simulink model "six_plus_six_AcmsteeringV09_main"  (R2014a)
settings: Solver=FixedStepDiscrete  StartTime=0.0  StopTime=10.0  FixedStep=0.0005  RelTol=1e-3
InitFcn:
  | Veh_Par_wxt
values from neighbouring files (symbols this model uses):
  acc_spdctl = [0 100]    [Veh_Par_wxt.m]
  ag_thr = ecucoder_cal(ag_thr)    [Veh_Par_wxt.m]
  B = 1.8    [Veh_Par_wxt.m]
  bra_em = 100    [Veh_Par_wxt.m]
  bra_pre_gz2 = 100/3    (= 33.3333333333)    [Veh_Par_wxt.m]
  bra_pre_gz34 = 10/3    (= 3.33333333333)    [Veh_Par_wxt.m]
  bra_pre_yd = 10/2    (= 5)    [Veh_Par_wxt.m]
  brakepre_dem_data = [0 1 2 3 4 5 6 7 8 9 10]    [Veh_Par_wxt.m]
  brakeTrq_dem_data = [0 125 251 376 502 627 753 878 1004 1129 1255]    [Veh_Par_wxt.m]
  bratrq_max = 4*1255    (= 5020)    [Veh_Par_wxt.m]
  eff_tran = 0.9    [Veh_Par_wxt.m]
  ESP_switch = ecucoder_cal(ESP_switch)    [Veh_Par_wxt.m]
  G = Mass*g    (= 15696)    [Veh_Par_wxt.m]
  kd1 = ecucoder_cal(kd1)    [Veh_Par_wxt.m]
  kd2 = 0    [Veh_Par_wxt.m]
  ki1 = ecucoder_cal(ki1)    [Veh_Par_wxt.m]
  ki2 = 1    [Veh_Par_wxt.m]
  kp1 = ecucoder_cal(kp1)    [Veh_Par_wxt.m]
  kp2 = 300    [Veh_Par_wxt.m]
  L = L1+L2    (= 2.9)    [Veh_Par_wxt.m]
  premax = 100    [Veh_Par_wxt.m]
  Radius = 0.4572/2    (= 0.2286)    [Veh_Par_wxt.m]
  RC_switch = ecucoder_cal(RC_switch)    [Veh_Par_wxt.m]
  s_opt_yi = 0.15    [Veh_Par_wxt.m]
  s_opt_zhuan = 0.8    [Veh_Par_wxt.m]
  s_opt_zhuan_add = 0.05    [Veh_Par_wxt.m]
  s_opt_zhuan_table = [0.8 0.8 0.3 0.3]    [Veh_Par_wxt.m]
  spd_map_mot = [0 499.85 999.79 1500 2000 2500 3000 3500 4000 4500 4999.8 5999.8]    [Veh_Par_wxt.m]
  spd_spdctl = [0 500]    [Veh_Par_wxt.m]
  speed_thr_park = 5/3.6/Radius*tras_ratio*30/pi    (= 464.143899364)    [Veh_Par_wxt.m]
  TCS_switch = ecucoder_cal(TCS_switch)    [Veh_Par_wxt.m]
  tras_ratio = 8    [Veh_Par_wxt.m]
  trq_map_mot = [70.5 70.012 71.154 65.797 53.917 45.159 38.073 32.685 27.48 17.133 14.949 10.07]    [Veh_Par_wxt.m]
  trqmax_yd = 70.5    [Veh_Par_wxt.m]
  trqmax_zx = 70.5    [Veh_Par_wxt.m]
  trqmaxneg = -70.5    [Veh_Par_wxt.m]
  v_gain = 0.9    [Veh_Par_wxt.m]
  v_table = [0 5 20 100]    [Veh_Par_wxt.m]
  v_thr_park = 5    [Veh_Par_wxt.m]
  zhidong_bianmazhi = [-140000 750000]    [Veh_Par_wxt.m]
  zhidong_down = -140000    [Veh_Par_wxt.m]
  zhidong_up = 750000    [Veh_Par_wxt.m]
  zhidong_youmen = [0 100]    [Veh_Par_wxt.m]
  zhuanxiang_bianmazhi = [-400000 0 400000]    [Veh_Par_wxt.m]
  zhuanxiang_down = -400000    [Veh_Par_wxt.m]
  zhuanxiang_up = 400000    [Veh_Par_wxt.m]
  zhuanxiang_youmen = [-100 0 100]    [Veh_Par_wxt.m]
undefined symbols (not defined in the file or in its folder): ecucoder_acal, guzhang_lf, guzhang_lm, guzhang_lr, guzhang_rf, guzhang_rm, guzhang_rr, myFIS
libraries: simulink x979, ec5744lib x59, fuzblock x2
(part 15 of 26)

== system six_plus_six_AcmsteeringV09_main/MainControl/mode_control/center_steer ==
  Signals : Inport
  Action Port : ActionPort  ActionType=case
  Mux : Mux  Inputs=10
  center_steer : Subsystem
  center_steer_dem : Outport
  wires:
  Mux/1 -> center_steer_dem/1
  Signals/1 -> center_steer/1(Signals)
  center_steer/6(mot_rr) -> Mux/6
  center_steer/1(mot_lf) -> Mux/1
  center_steer/4(mot_rf) -> Mux/4
  center_steer/3(mot_lr) -> Mux/3
  center_steer/5(mot_rm) -> Mux/5
  center_steer/2(mot_lm) -> Mux/2
  center_steer/7(motec_position_1) -> Mux/7
  center_steer/8(motec_position_2) -> Mux/8
  center_steer/10(motec_position_4) -> Mux/10
  center_steer/9(motec_position_3) -> Mux/9

== system six_plus_six_AcmsteeringV09_main/MainControl/mode_control/emergency_stop ==
  Signals : Inport
  Action Port : ActionPort  ActionType=case
  Mux : Mux  Inputs=10
  emergency_stop : Subsystem
  emergency_stop_dem : Outport
  wires:
  Mux/1 -> emergency_stop_dem/1
  Signals/1 -> emergency_stop/1(Signals)
  emergency_stop/8(motec_position_2) -> Mux/8
  emergency_stop/9(motec_position_3) -> Mux/9
  emergency_stop/10(motec_position_4) -> Mux/10
  emergency_stop/7(motec_position_1) -> Mux/7
  emergency_stop/3(mot_lr) -> Mux/3
  emergency_stop/1(mot_lf) -> Mux/1
  emergency_stop/2(mot_lm) -> Mux/2
  emergency_stop/5(mot_rm) -> Mux/5
  emergency_stop/6(mot_rr) -> Mux/6
  emergency_stop/4(mot_rf) -> Mux/4

== system six_plus_six_AcmsteeringV09_main/MainControl/mode_control/forward ==
  Signals : Inport
  Action Port : ActionPort  ActionType=case
  forward : Subsystem
  forward_dem : Outport
  wires:
  Signals/1 -> forward/1(Signals)
  forward/1(forward_dem) -> forward_dem/1

== system six_plus_six_AcmsteeringV09_main/MainControl/mode_control/neutral ==
  Signals : Inport
  Action Port : ActionPort  ActionType=case
  Mux : Mux  Inputs=10
  neutral : Subsystem
  neutral_dem : Outport
  wires:
  Mux/1 -> neutral_dem/1
  Signals/1 -> neutral/1(Signals)
  neutral/3(mot_lr) -> Mux/3
  neutral/5(mot_rm) -> Mux/5
  neutral/6(mot_rr) -> Mux/6
  neutral/2(mot_lm) -> Mux/2
  neutral/1(mot_lf) -> Mux/1
  neutral/4(mot_rf) -> Mux/4
  neutral/7(motec_position_1) -> Mux/7
  neutral/8(motec_position_2) -> Mux/8
  neutral/10(motec_position_4) -> Mux/10
  neutral/9(motec_position_3) -> Mux/9

== system six_plus_six_AcmsteeringV09_main/Subsystem/VCU1/VCU1_CtrlModel ==
  VCU1_CtrlModel : Inport
  Constant{2..8} (7 alike) : Constant  Value=0  OutDataTypeStr=uint8
  VCU1_CtrlModelRon : Rounding  Operator=round
  VCU1_CtrlModel_1sat : Saturate  UpperLimit=4  LowerLimit=0
  VCU1_CtrlModel_Convert : DataTypeConversion  OutDataTypeStr=uint8
  VCU1_CtrlModel_Convert1 : DataTypeConversion  OutDataTypeStr=uint32
  VCU1_CtrlModel_D : Product  Inputs=*/
  VCU1_CtrlModel_F : Constant  OutDataTypeStr=single
  VCU1_CtrlModel_L : simulink/Logic and Bit Operations/Bitwise Operator  logicop=AND  UseBitMask=on  BitMask=4  BitMaskRealWorld=Stored Integer
  VCU1_CtrlModel_O : Constant  Value=0  OutDataTypeStr=single
  VCU1_CtrlModel_S : ArithShift  BitShiftNumber=-2
  VCU1_CtrlModel_sat : Saturate  UpperLimit=1  LowerLimit=0
  VCU1_CtrlModel_st : Sum  Inputs=+-
  output1 : Outport
  output2 : Outport  Port=2
  output3 : Outport  Port=3
  output4 : Outport  Port=4
  output5 : Outport  Port=5
  output6 : Outport  Port=6
  output7 : Outport  Port=7
  output8 : Outport  Port=8
  wires:
  VCU1_CtrlModel/1 -> VCU1_CtrlModel_sat/1
  VCU1_CtrlModel_sat/1 -> VCU1_CtrlModel_st/1
  VCU1_CtrlModel_O/1 -> VCU1_CtrlModel_st/2
  VCU1_CtrlModel_st/1 -> VCU1_CtrlModel_D/1
  VCU1_CtrlModel_F/1 -> VCU1_CtrlModel_D/2
  VCU1_CtrlModel_D/1 -> VCU1_CtrlModelRon/1
  VCU1_CtrlModelRon/1 -> VCU1_CtrlModel_S/1
  VCU1_CtrlModel_S/1 -> VCU1_CtrlModel_1sat/1
  VCU1_CtrlModel_1sat/1 -> VCU1_CtrlModel_Convert1/1
  VCU1_CtrlModel_Convert1/1 -> VCU1_CtrlModel_L/1
  VCU1_CtrlModel_L/1 -> VCU1_CtrlModel_Convert/1
  VCU1_CtrlModel_Convert/1 -> output1/1
  Constant2/1 -> output2/1
  Constant3/1 -> output3/1
  Constant4/1 -> output4/1
  Constant5/1 -> output5/1
  Constant6/1 -> output6/1
  Constant7/1 -> output7/1
  Constant8/1 -> output8/1

== system six_plus_six_AcmsteeringV09_main/Subsystem/VCU1/VCU1_EnableReq ==
  VCU1_EnableReq : Inport
  Constant{2..8} (7 alike) : Constant  Value=0  OutDataTypeStr=uint8
  VCU1_EnableReqRon : Rounding  Operator=round
  VCU1_EnableReq_1sat : Saturate  UpperLimit=3  LowerLimit=0
  VCU1_EnableReq_Convert : DataTypeConversion  OutDataTypeStr=uint8
  VCU1_EnableReq_Convert1 : DataTypeConversion  OutDataTypeStr=uint32
  VCU1_EnableReq_D : Product  Inputs=*/
  VCU1_EnableReq_F : Constant  OutDataTypeStr=single
  VCU1_EnableReq_L : simulink/Logic and Bit Operations/Bitwise Operator  logicop=AND  UseBitMask=on  BitMask=3  BitMaskRealWorld=Stored Integer
  VCU1_EnableReq_O : Constant  Value=0  OutDataTypeStr=single
  VCU1_EnableReq_S : ArithShift
  VCU1_EnableReq_sat : Saturate  UpperLimit=3  LowerLimit=0
  VCU1_EnableReq_st : Sum  Inputs=+-
  output1 : Outport
  output2 : Outport  Port=2
  output3 : Outport  Port=3
  output4 : Outport  Port=4
  output5 : Outport  Port=5
  output6 : Outport  Port=6
  output7 : Outport  Port=7
  output8 : Outport  Port=8
  wires:
  VCU1_EnableReq/1 -> VCU1_EnableReq_sat/1
  VCU1_EnableReq_sat/1 -> VCU1_EnableReq_st/1
  VCU1_EnableReq_O/1 -> VCU1_EnableReq_st/2
  VCU1_EnableReq_st/1 -> VCU1_EnableReq_D/1
  VCU1_EnableReq_F/1 -> VCU1_EnableReq_D/2
  VCU1_EnableReq_D/1 -> VCU1_EnableReqRon/1
  VCU1_EnableReqRon/1 -> VCU1_EnableReq_S/1
  VCU1_EnableReq_S/1 -> VCU1_EnableReq_1sat/1
  VCU1_EnableReq_1sat/1 -> VCU1_EnableReq_Convert1/1
  VCU1_EnableReq_Convert1/1 -> VCU1_EnableReq_L/1
  VCU1_EnableReq_L/1 -> VCU1_EnableReq_Convert/1
  VCU1_EnableReq_Convert/1 -> output1/1
  Constant2/1 -> output2/1
  Constant3/1 -> output3/1
  Constant4/1 -> output4/1
  Constant5/1 -> output5/1
  Constant6/1 -> output6/1
  Constant7/1 -> output7/1
  Constant8/1 -> output8/1

== system six_plus_six_AcmsteeringV09_main/Subsystem/VCU1/VCU1_GearCmd ==
  VCU1_GearCmd : Inport
  Constant{2..8} (7 alike) : Constant  Value=0  OutDataTypeStr=uint8
  VCU1_GearCmdRon : Rounding  Operator=round
  VCU1_GearCmd_1sat : Saturate  UpperLimit=24  LowerLimit=0
  VCU1_GearCmd_Convert : DataTypeConversion  OutDataTypeStr=uint8
  VCU1_GearCmd_Convert1 : DataTypeConversion  OutDataTypeStr=uint32
  VCU1_GearCmd_D : Product  Inputs=*/
  VCU1_GearCmd_F : Constant  OutDataTypeStr=single
  VCU1_GearCmd_L : simulink/Logic and Bit Operations/Bitwise Operator  logicop=AND  UseBitMask=on  BitMask=24  BitMaskRealWorld=Stored Integer
  VCU1_GearCmd_O : Constant  Value=0  OutDataTypeStr=single
  VCU1_GearCmd_S : ArithShift  BitShiftNumber=-3
  VCU1_GearCmd_sat : Saturate  UpperLimit=3  LowerLimit=0
  VCU1_GearCmd_st : Sum  Inputs=+-
  output1 : Outport
  output2 : Outport  Port=2
  output3 : Outport  Port=3
  output4 : Outport  Port=4
  output5 : Outport  Port=5
  output6 : Outport  Port=6
  output7 : Outport  Port=7
  output8 : Outport  Port=8
  wires:
  VCU1_GearCmd/1 -> VCU1_GearCmd_sat/1
  VCU1_GearCmd_sat/1 -> VCU1_GearCmd_st/1
  VCU1_GearCmd_O/1 -> VCU1_GearCmd_st/2
  VCU1_GearCmd_st/1 -> VCU1_GearCmd_D/1
  VCU1_GearCmd_F/1 -> VCU1_GearCmd_D/2
  VCU1_GearCmd_D/1 -> VCU1_GearCmdRon/1
  VCU1_GearCmdRon/1 -> VCU1_GearCmd_S/1
  VCU1_GearCmd_S/1 -> VCU1_GearCmd_1sat/1
  VCU1_GearCmd_1sat/1 -> VCU1_GearCmd_Convert1/1
  VCU1_GearCmd_Convert1/1 -> VCU1_GearCmd_L/1
  VCU1_GearCmd_L/1 -> VCU1_GearCmd_Convert/1
  VCU1_GearCmd_Convert/1 -> output1/1
  Constant2/1 -> output2/1
  Constant3/1 -> output3/1
  Constant4/1 -> output4/1
  Constant5/1 -> output5/1
  Constant6/1 -> output6/1
  Constant7/1 -> output7/1
  Constant8/1 -> output8/1

== system six_plus_six_AcmsteeringV09_main/Subsystem/VCU1/VCU1_LifeCnt ==
  VCU1_LifeCnt : Inport
  Constant{1..7} (7 alike) : Constant  Value=0  OutDataTypeStr=uint8
  VCU1_LifeCntRon : Rounding  Operator=round
  VCU1_LifeCnt_1sat : Saturate  UpperLimit=255  LowerLimit=0
  VCU1_LifeCnt_Convert : DataTypeConversion  OutDataTypeStr=uint8
  VCU1_LifeCnt_Convert1 : DataTypeConversion  OutDataTypeStr=uint32
  VCU1_LifeCnt_D : Product  Inputs=*/
  VCU1_LifeCnt_F : Constant  OutDataTypeStr=single
  VCU1_LifeCnt_L : simulink/Logic and Bit Operations/Bitwise Operator  logicop=AND  UseBitMask=on  BitMask=255  BitMaskRealWorld=Stored Integer
  VCU1_LifeCnt_O : Constant  Value=0  OutDataTypeStr=single
  VCU1_LifeCnt_S : ArithShift
  VCU1_LifeCnt_sat : Saturate  UpperLimit=255  LowerLimit=0
  VCU1_LifeCnt_st : Sum  Inputs=+-
  output1 : Outport
  output2 : Outport  Port=2
  output3 : Outport  Port=3
  output4 : Outport  Port=4
  output5 : Outport  Port=5
  output6 : Outport  Port=6
  output7 : Outport  Port=7
  output8 : Outport  Port=8
  wires:
  VCU1_LifeCnt/1 -> VCU1_LifeCnt_sat/1
  VCU1_LifeCnt_sat/1 -> VCU1_LifeCnt_st/1
  VCU1_LifeCnt_O/1 -> VCU1_LifeCnt_st/2
  VCU1_LifeCnt_st/1 -> VCU1_LifeCnt_D/1
  VCU1_LifeCnt_F/1 -> VCU1_LifeCnt_D/2
  VCU1_LifeCnt_D/1 -> VCU1_LifeCntRon/1
  VCU1_LifeCntRon/1 -> VCU1_LifeCnt_S/1
  VCU1_LifeCnt_S/1 -> VCU1_LifeCnt_1sat/1
  VCU1_LifeCnt_1sat/1 -> VCU1_LifeCnt_Convert1/1
  VCU1_LifeCnt_Convert1/1 -> VCU1_LifeCnt_L/1
  VCU1_LifeCnt_L/1 -> VCU1_LifeCnt_Convert/1
  VCU1_LifeCnt_Convert/1 -> output8/1
  Constant1/1 -> output1/1
  Constant2/1 -> output2/1
  Constant3/1 -> output3/1
  Constant4/1 -> output4/1
  Constant5/1 -> output5/1
  Constant6/1 -> output6/1
  Constant7/1 -> output7/1

== system six_plus_six_AcmsteeringV09_main/Subsystem/VCU1/VCU1_SpeedMax ==
  VCU1_SpeedMax : Inport
  Constant{1,4..8} (6 alike) : Constant  Value=0  OutDataTypeStr=uint8
  VCU1_SpeedMaxBitCov : DataTypeConversion  OutDataTypeStr=uint8
  VCU1_SpeedMaxCOV : DataTypeConversion  OutDataTypeStr=uint8
  VCU1_SpeedMaxRon : Rounding  Operator=round
  VCU1_SpeedMax_1sat : Saturate  UpperLimit=65535  LowerLimit=0
  VCU1_SpeedMax_And : simulink/Logic and Bit Operations/Bitwise Operator  logicop=AND  UseBitMask=off  NumInputPorts=2  BitMask=bin2dec('11011001')  BitMaskRealWorld=Stored Integer
  VCU1_SpeedMax_And_C : Constant  Value=255  OutDataTypeStr=uint32
  VCU1_SpeedMax_Convert : DataTypeConversion  OutDataTypeStr=uint32
  VCU1_SpeedMax_D : Product  Inputs=*/
  VCU1_SpeedMax_D1 : Product  Inputs=*/
  VCU1_SpeedMax_F : Constant  OutDataTypeStr=single
  VCU1_SpeedMax_L : simulink/Logic and Bit Operations/Bitwise Operator  logicop=AND  UseBitMask=on  BitMask=65535  BitMaskRealWorld=Stored Integer
  VCU1_SpeedMax_O : Constant  Value=0  OutDataTypeStr=single
  VCU1_SpeedMax_S : ArithShift
  VCU1_SpeedMax_sat : Saturate  UpperLimit=10000  LowerLimit=0
  VCU1_SpeedMax_st : Sum  Inputs=+-
  VCU1_SpeedMaxoutput2_C : Constant  Value=256
  output1 : Outport
  output2 : Outport  Port=2
  output3 : Outport  Port=3
  output4 : Outport  Port=4
  output5 : Outport  Port=5
  output6 : Outport  Port=6
  output7 : Outport  Port=7
  output8 : Outport  Port=8
  wires:
  VCU1_SpeedMax/1 -> VCU1_SpeedMax_sat/1
  VCU1_SpeedMax_sat/1 -> VCU1_SpeedMax_st/1
  VCU1_SpeedMax_O/1 -> VCU1_SpeedMax_st/2
  VCU1_SpeedMax_st/1 -> VCU1_SpeedMax_D/1
  VCU1_SpeedMax_F/1 -> VCU1_SpeedMax_D/2
  VCU1_SpeedMax_D/1 -> VCU1_SpeedMaxRon/1
  VCU1_SpeedMaxRon/1 -> VCU1_SpeedMax_S/1
  VCU1_SpeedMax_S/1 -> VCU1_SpeedMax_1sat/1
  VCU1_SpeedMax_1sat/1 -> VCU1_SpeedMax_Convert/1
  VCU1_SpeedMax_Convert/1 -> VCU1_SpeedMax_L/1
  VCU1_SpeedMax_L/1 -> VCU1_SpeedMax_D1/1, VCU1_SpeedMax_And/1
  VCU1_SpeedMaxoutput2_C/1 -> VCU1_SpeedMax_D1/2
  VCU1_SpeedMax_D1/1 -> VCU1_SpeedMaxCOV/1
  VCU1_SpeedMaxCOV/1 -> output2/1
  VCU1_SpeedMax_And_C/1 -> VCU1_SpeedMax_And/2
  VCU1_SpeedMax_And/1 -> VCU1_SpeedMaxBitCov/1
  VCU1_SpeedMaxBitCov/1 -> output3/1
  Constant1/1 -> output1/1
  Constant4/1 -> output4/1
  Constant5/1 -> output5/1
  Constant6/1 -> output6/1
  Constant7/1 -> output7/1
  Constant8/1 -> output8/1

== system six_plus_six_AcmsteeringV09_main/Subsystem/VCU1/VCU1_TorqueRef ==
  VCU1_TorqueRef : Inport
  Constant{1..3,6..8} (6 alike) : Constant  Value=0  OutDataTypeStr=uint8
  VCU1_TorqueRefBitCov : DataTypeConversion  OutDataTypeStr=uint8
  VCU1_TorqueRefCOV : DataTypeConversion  OutDataTypeStr=uint8
  VCU1_TorqueRefRon : Rounding  Operator=round
  VCU1_TorqueRef_1sat : Saturate  UpperLimit=65535  LowerLimit=0
  VCU1_TorqueRef_And : simulink/Logic and Bit Operations/Bitwise Operator  logicop=AND  UseBitMask=off  NumInputPorts=2  BitMask=bin2dec('11011001')  BitMaskRealWorld=Stored Integer
  VCU1_TorqueRef_And_C : Constant  Value=255  OutDataTypeStr=uint32
  VCU1_TorqueRef_Convert : DataTypeConversion  OutDataTypeStr=uint32
  VCU1_TorqueRef_D : Product  Inputs=*/
  VCU1_TorqueRef_D1 : Product  Inputs=*/
  VCU1_TorqueRef_F : Constant  Value=0.1  OutDataTypeStr=single
  VCU1_TorqueRef_L : simulink/Logic and Bit Operations/Bitwise Operator  logicop=AND  UseBitMask=on  BitMask=65535  BitMaskRealWorld=Stored Integer
  VCU1_TorqueRef_O : Constant  Value=-1000  OutDataTypeStr=single
  VCU1_TorqueRef_S : ArithShift
  VCU1_TorqueRef_sat : Saturate  UpperLimit=1000  LowerLimit=-1000
  VCU1_TorqueRef_st : Sum  Inputs=+-
  VCU1_TorqueRefoutput4_C : Constant  Value=256
  output1 : Outport
  output2 : Outport  Port=2
  output3 : Outport  Port=3
  output4 : Outport  Port=4
  output5 : Outport  Port=5
  output6 : Outport  Port=6
  output7 : Outport  Port=7
  output8 : Outport  Port=8
  wires:
  VCU1_TorqueRef/1 -> VCU1_TorqueRef_sat/1
  VCU1_TorqueRef_sat/1 -> VCU1_TorqueRef_st/1
  VCU1_TorqueRef_O/1 -> VCU1_TorqueRef_st/2
  VCU1_TorqueRef_st/1 -> VCU1_TorqueRef_D/1
  VCU1_TorqueRef_F/1 -> VCU1_TorqueRef_D/2
  VCU1_TorqueRef_D/1 -> VCU1_TorqueRefRon/1
  VCU1_TorqueRefRon/1 -> VCU1_TorqueRef_S/1
  VCU1_TorqueRef_S/1 -> VCU1_TorqueRef_1sat/1
  VCU1_TorqueRef_1sat/1 -> VCU1_TorqueRef_Convert/1
  VCU1_TorqueRef_Convert/1 -> VCU1_TorqueRef_L/1
  VCU1_TorqueRef_L/1 -> VCU1_TorqueRef_D1/1, VCU1_TorqueRef_And/1
  VCU1_TorqueRefoutput4_C/1 -> VCU1_TorqueRef_D1/2
  VCU1_TorqueRef_D1/1 -> VCU1_TorqueRefCOV/1
  VCU1_TorqueRefCOV/1 -> output4/1
  VCU1_TorqueRef_And_C/1 -> VCU1_TorqueRef_And/2
  VCU1_TorqueRef_And/1 -> VCU1_TorqueRefBitCov/1
  VCU1_TorqueRefBitCov/1 -> output5/1
  Constant1/1 -> output1/1
  Constant2/1 -> output2/1
  Constant3/1 -> output3/1
  Constant6/1 -> output6/1
  Constant7/1 -> output7/1
  Constant8/1 -> output8/1

== system six_plus_six_AcmsteeringV09_main/Subsystem/VCU2/VCU1_CtrlModel ==
  VCU1_CtrlModel : Inport
  Constant{2..8} (7 alike) : Constant  Value=0  OutDataTypeStr=uint8
  VCU1_CtrlModelRon : Rounding  Operator=round
  VCU1_CtrlModel_1sat : Saturate  UpperLimit=4  LowerLimit=0
  VCU1_CtrlModel_Convert : DataTypeConversion  OutDataTypeStr=uint8
  VCU1_CtrlModel_Convert1 : DataTypeConversion  OutDataTypeStr=uint32
  VCU1_CtrlModel_D : Product  Inputs=*/
  VCU1_CtrlModel_F : Constant  OutDataTypeStr=single
  VCU1_CtrlModel_L : simulink/Logic and Bit Operations/Bitwise Operator  logicop=AND  UseBitMask=on  BitMask=4  BitMaskRealWorld=Stored Integer
  VCU1_CtrlModel_O : Constant  Value=0  OutDataTypeStr=single
  VCU1_CtrlModel_S : ArithShift  BitShiftNumber=-2
  VCU1_CtrlModel_sat : Saturate  UpperLimit=1  LowerLimit=0
  VCU1_CtrlModel_st : Sum  Inputs=+-
  output1 : Outport
  output2 : Outport  Port=2
  output3 : Outport  Port=3
  output4 : Outport  Port=4
  output5 : Outport  Port=5
  output6 : Outport  Port=6
  output7 : Outport  Port=7
  output8 : Outport  Port=8
  wires:
  VCU1_CtrlModel/1 -> VCU1_CtrlModel_sat/1
  VCU1_CtrlModel_sat/1 -> VCU1_CtrlModel_st/1
  VCU1_CtrlModel_O/1 -> VCU1_CtrlModel_st/2
  VCU1_CtrlModel_st/1 -> VCU1_CtrlModel_D/1
  VCU1_CtrlModel_F/1 -> VCU1_CtrlModel_D/2
  VCU1_CtrlModel_D/1 -> VCU1_CtrlModelRon/1
  VCU1_CtrlModelRon/1 -> VCU1_CtrlModel_S/1
  VCU1_CtrlModel_S/1 -> VCU1_CtrlModel_1sat/1
  VCU1_CtrlModel_1sat/1 -> VCU1_CtrlModel_Convert1/1
  VCU1_CtrlModel_Convert1/1 -> VCU1_CtrlModel_L/1
  VCU1_CtrlModel_L/1 -> VCU1_CtrlModel_Convert/1
  VCU1_CtrlModel_Convert/1 -> output1/1
  Constant2/1 -> output2/1
  Constant3/1 -> output3/1
  Constant4/1 -> output4/1
  Constant5/1 -> output5/1
  Constant6/1 -> output6/1
  Constant7/1 -> output7/1
  Constant8/1 -> output8/1

== system six_plus_six_AcmsteeringV09_main/Subsystem/VCU2/VCU1_EnableReq ==
  VCU1_EnableReq : Inport
  Constant{2..8} (7 alike) : Constant  Value=0  OutDataTypeStr=uint8
  VCU1_EnableReqRon : Rounding  Operator=round
  VCU1_EnableReq_1sat : Saturate  UpperLimit=3  LowerLimit=0
  VCU1_EnableReq_Convert : DataTypeConversion  OutDataTypeStr=uint8
  VCU1_EnableReq_Convert1 : DataTypeConversion  OutDataTypeStr=uint32
  VCU1_EnableReq_D : Product  Inputs=*/
  VCU1_EnableReq_F : Constant  OutDataTypeStr=single
  VCU1_EnableReq_L : simulink/Logic and Bit Operations/Bitwise Operator  logicop=AND  UseBitMask=on  BitMask=3  BitMaskRealWorld=Stored Integer
  VCU1_EnableReq_O : Constant  Value=0  OutDataTypeStr=single
  VCU1_EnableReq_S : ArithShift
  VCU1_EnableReq_sat : Saturate  UpperLimit=3  LowerLimit=0
  VCU1_EnableReq_st : Sum  Inputs=+-
  output1 : Outport
  output2 : Outport  Port=2
  output3 : Outport  Port=3
  output4 : Outport  Port=4
  output5 : Outport  Port=5
  output6 : Outport  Port=6
  output7 : Outport  Port=7
  output8 : Outport  Port=8
  wires:
  VCU1_EnableReq/1 -> VCU1_EnableReq_sat/1
  VCU1_EnableReq_sat/1 -> VCU1_EnableReq_st/1
  VCU1_EnableReq_O/1 -> VCU1_EnableReq_st/2
  VCU1_EnableReq_st/1 -> VCU1_EnableReq_D/1
  VCU1_EnableReq_F/1 -> VCU1_EnableReq_D/2
  VCU1_EnableReq_D/1 -> VCU1_EnableReqRon/1
  VCU1_EnableReqRon/1 -> VCU1_EnableReq_S/1
  VCU1_EnableReq_S/1 -> VCU1_EnableReq_1sat/1
  VCU1_EnableReq_1sat/1 -> VCU1_EnableReq_Convert1/1
  VCU1_EnableReq_Convert1/1 -> VCU1_EnableReq_L/1
  VCU1_EnableReq_L/1 -> VCU1_EnableReq_Convert/1
  VCU1_EnableReq_Convert/1 -> output1/1
  Constant2/1 -> output2/1
  Constant3/1 -> output3/1
  Constant4/1 -> output4/1
  Constant5/1 -> output5/1
  Constant6/1 -> output6/1
  Constant7/1 -> output7/1
  Constant8/1 -> output8/1

== system six_plus_six_AcmsteeringV09_main/Subsystem/VCU2/VCU1_GearCmd ==
  VCU1_GearCmd : Inport
  Constant{2..8} (7 alike) : Constant  Value=0  OutDataTypeStr=uint8
  VCU1_GearCmdRon : Rounding  Operator=round
  VCU1_GearCmd_1sat : Saturate  UpperLimit=24  LowerLimit=0
  VCU1_GearCmd_Convert : DataTypeConversion  OutDataTypeStr=uint8
  VCU1_GearCmd_Convert1 : DataTypeConversion  OutDataTypeStr=uint32
  VCU1_GearCmd_D : Product  Inputs=*/
  VCU1_GearCmd_F : Constant  OutDataTypeStr=single
  VCU1_GearCmd_L : simulink/Logic and Bit Operations/Bitwise Operator  logicop=AND  UseBitMask=on  BitMask=24  BitMaskRealWorld=Stored Integer
  VCU1_GearCmd_O : Constant  Value=0  OutDataTypeStr=single
  VCU1_GearCmd_S : ArithShift  BitShiftNumber=-3
  VCU1_GearCmd_sat : Saturate  UpperLimit=3  LowerLimit=0
  VCU1_GearCmd_st : Sum  Inputs=+-
  output1 : Outport
  output2 : Outport  Port=2
  output3 : Outport  Port=3
  output4 : Outport  Port=4
  output5 : Outport  Port=5
  output6 : Outport  Port=6
  output7 : Outport  Port=7
  output8 : Outport  Port=8
  wires:
  VCU1_GearCmd/1 -> VCU1_GearCmd_sat/1
  VCU1_GearCmd_sat/1 -> VCU1_GearCmd_st/1
  VCU1_GearCmd_O/1 -> VCU1_GearCmd_st/2
  VCU1_GearCmd_st/1 -> VCU1_GearCmd_D/1
  VCU1_GearCmd_F/1 -> VCU1_GearCmd_D/2
  VCU1_GearCmd_D/1 -> VCU1_GearCmdRon/1
  VCU1_GearCmdRon/1 -> VCU1_GearCmd_S/1
  VCU1_GearCmd_S/1 -> VCU1_GearCmd_1sat/1
  VCU1_GearCmd_1sat/1 -> VCU1_GearCmd_Convert1/1
  VCU1_GearCmd_Convert1/1 -> VCU1_GearCmd_L/1
  VCU1_GearCmd_L/1 -> VCU1_GearCmd_Convert/1
  VCU1_GearCmd_Convert/1 -> output1/1
  Constant2/1 -> output2/1
  Constant3/1 -> output3/1
  Constant4/1 -> output4/1
  Constant5/1 -> output5/1
  Constant6/1 -> output6/1
  Constant7/1 -> output7/1
  Constant8/1 -> output8/1

== system six_plus_six_AcmsteeringV09_main/Subsystem/VCU2/VCU1_LifeCnt ==
  VCU1_LifeCnt : Inport
  Constant{1..7} (7 alike) : Constant  Value=0  OutDataTypeStr=uint8
  VCU1_LifeCntRon : Rounding  Operator=round
  VCU1_LifeCnt_1sat : Saturate  UpperLimit=255  LowerLimit=0
  VCU1_LifeCnt_Convert : DataTypeConversion  OutDataTypeStr=uint8
  VCU1_LifeCnt_Convert1 : DataTypeConversion  OutDataTypeStr=uint32
  VCU1_LifeCnt_D : Product  Inputs=*/
  VCU1_LifeCnt_F : Constant  OutDataTypeStr=single
  VCU1_LifeCnt_L : simulink/Logic and Bit Operations/Bitwise Operator  logicop=AND  UseBitMask=on  BitMask=255  BitMaskRealWorld=Stored Integer
  VCU1_LifeCnt_O : Constant  Value=0  OutDataTypeStr=single
  VCU1_LifeCnt_S : ArithShift
  VCU1_LifeCnt_sat : Saturate  UpperLimit=255  LowerLimit=0
  VCU1_LifeCnt_st : Sum  Inputs=+-
  output1 : Outport
  output2 : Outport  Port=2
  output3 : Outport  Port=3
  output4 : Outport  Port=4
  output5 : Outport  Port=5
  output6 : Outport  Port=6
  output7 : Outport  Port=7
  output8 : Outport  Port=8
  wires:
  VCU1_LifeCnt/1 -> VCU1_LifeCnt_sat/1
  VCU1_LifeCnt_sat/1 -> VCU1_LifeCnt_st/1
  VCU1_LifeCnt_O/1 -> VCU1_LifeCnt_st/2
  VCU1_LifeCnt_st/1 -> VCU1_LifeCnt_D/1
  VCU1_LifeCnt_F/1 -> VCU1_LifeCnt_D/2
  VCU1_LifeCnt_D/1 -> VCU1_LifeCntRon/1
  VCU1_LifeCntRon/1 -> VCU1_LifeCnt_S/1
  VCU1_LifeCnt_S/1 -> VCU1_LifeCnt_1sat/1
  VCU1_LifeCnt_1sat/1 -> VCU1_LifeCnt_Convert1/1
  VCU1_LifeCnt_Convert1/1 -> VCU1_LifeCnt_L/1
  VCU1_LifeCnt_L/1 -> VCU1_LifeCnt_Convert/1
  VCU1_LifeCnt_Convert/1 -> output8/1
  Constant1/1 -> output1/1
  Constant2/1 -> output2/1
  Constant3/1 -> output3/1
  Constant4/1 -> output4/1
  Constant5/1 -> output5/1
  Constant6/1 -> output6/1
  Constant7/1 -> output7/1

== system six_plus_six_AcmsteeringV09_main/Subsystem/VCU2/VCU1_SpeedMax ==
  VCU1_SpeedMax : Inport
  Constant{1,4..8} (6 alike) : Constant  Value=0  OutDataTypeStr=uint8
  VCU1_SpeedMaxBitCov : DataTypeConversion  OutDataTypeStr=uint8
  VCU1_SpeedMaxCOV : DataTypeConversion  OutDataTypeStr=uint8
  VCU1_SpeedMaxRon : Rounding  Operator=round
  VCU1_SpeedMax_1sat : Saturate  UpperLimit=65535  LowerLimit=0
  VCU1_SpeedMax_And : simulink/Logic and Bit Operations/Bitwise Operator  logicop=AND  UseBitMask=off  NumInputPorts=2  BitMask=bin2dec('11011001')  BitMaskRealWorld=Stored Integer
  VCU1_SpeedMax_And_C : Constant  Value=255  OutDataTypeStr=uint32
  VCU1_SpeedMax_Convert : DataTypeConversion  OutDataTypeStr=uint32
  VCU1_SpeedMax_D : Product  Inputs=*/
  VCU1_SpeedMax_D1 : Product  Inputs=*/
  VCU1_SpeedMax_F : Constant  OutDataTypeStr=single
  VCU1_SpeedMax_L : simulink/Logic and Bit Operations/Bitwise Operator  logicop=AND  UseBitMask=on  BitMask=65535  BitMaskRealWorld=Stored Integer
  VCU1_SpeedMax_O : Constant  Value=0  OutDataTypeStr=single
  VCU1_SpeedMax_S : ArithShift
  VCU1_SpeedMax_sat : Saturate  UpperLimit=10000  LowerLimit=0
  VCU1_SpeedMax_st : Sum  Inputs=+-
  VCU1_SpeedMaxoutput2_C : Constant  Value=256
  output1 : Outport
  output2 : Outport  Port=2
  output3 : Outport  Port=3
  output4 : Outport  Port=4
  output5 : Outport  Port=5
  output6 : Outport  Port=6
  output7 : Outport  Port=7
  output8 : Outport  Port=8
  wires:
  VCU1_SpeedMax/1 -> VCU1_SpeedMax_sat/1
  VCU1_SpeedMax_sat/1 -> VCU1_SpeedMax_st/1
  VCU1_SpeedMax_O/1 -> VCU1_SpeedMax_st/2
  VCU1_SpeedMax_st/1 -> VCU1_SpeedMax_D/1
  VCU1_SpeedMax_F/1 -> VCU1_SpeedMax_D/2
  VCU1_SpeedMax_D/1 -> VCU1_SpeedMaxRon/1
  VCU1_SpeedMaxRon/1 -> VCU1_SpeedMax_S/1
  VCU1_SpeedMax_S/1 -> VCU1_SpeedMax_1sat/1
  VCU1_SpeedMax_1sat/1 -> VCU1_SpeedMax_Convert/1
  VCU1_SpeedMax_Convert/1 -> VCU1_SpeedMax_L/1
  VCU1_SpeedMax_L/1 -> VCU1_SpeedMax_D1/1, VCU1_SpeedMax_And/1
  VCU1_SpeedMaxoutput2_C/1 -> VCU1_SpeedMax_D1/2
  VCU1_SpeedMax_D1/1 -> VCU1_SpeedMaxCOV/1
  VCU1_SpeedMaxCOV/1 -> output2/1
  VCU1_SpeedMax_And_C/1 -> VCU1_SpeedMax_And/2
  VCU1_SpeedMax_And/1 -> VCU1_SpeedMaxBitCov/1
  VCU1_SpeedMaxBitCov/1 -> output3/1
  Constant1/1 -> output1/1
  Constant4/1 -> output4/1
  Constant5/1 -> output5/1
  Constant6/1 -> output6/1
  Constant7/1 -> output7/1
  Constant8/1 -> output8/1

== system six_plus_six_AcmsteeringV09_main/Subsystem/VCU2/VCU1_TorqueRef ==
  VCU1_TorqueRef : Inport
  Constant{1..3,6..8} (6 alike) : Constant  Value=0  OutDataTypeStr=uint8
  VCU1_TorqueRefBitCov : DataTypeConversion  OutDataTypeStr=uint8
  VCU1_TorqueRefCOV : DataTypeConversion  OutDataTypeStr=uint8
  VCU1_TorqueRefRon : Rounding  Operator=round
  VCU1_TorqueRef_1sat : Saturate  UpperLimit=65535  LowerLimit=0
  VCU1_TorqueRef_And : simulink/Logic and Bit Operations/Bitwise Operator  logicop=AND  UseBitMask=off  NumInputPorts=2  BitMask=bin2dec('11011001')  BitMaskRealWorld=Stored Integer
  VCU1_TorqueRef_And_C : Constant  Value=255  OutDataTypeStr=uint32
  VCU1_TorqueRef_Convert : DataTypeConversion  OutDataTypeStr=uint32
  VCU1_TorqueRef_D : Product  Inputs=*/
  VCU1_TorqueRef_D1 : Product  Inputs=*/
  VCU1_TorqueRef_F : Constant  Value=0.1  OutDataTypeStr=single
  VCU1_TorqueRef_L : simulink/Logic and Bit Operations/Bitwise Operator  logicop=AND  UseBitMask=on  BitMask=65535  BitMaskRealWorld=Stored Integer
  VCU1_TorqueRef_O : Constant  Value=-1000  OutDataTypeStr=single
  VCU1_TorqueRef_S : ArithShift
  VCU1_TorqueRef_sat : Saturate  UpperLimit=1000  LowerLimit=-1000
  VCU1_TorqueRef_st : Sum  Inputs=+-
  VCU1_TorqueRefoutput4_C : Constant  Value=256
  output1 : Outport
  output2 : Outport  Port=2
  output3 : Outport  Port=3
  output4 : Outport  Port=4
  output5 : Outport  Port=5
  output6 : Outport  Port=6
  output7 : Outport  Port=7
  output8 : Outport  Port=8
  wires:
  VCU1_TorqueRef/1 -> VCU1_TorqueRef_sat/1
  VCU1_TorqueRef_sat/1 -> VCU1_TorqueRef_st/1
  VCU1_TorqueRef_O/1 -> VCU1_TorqueRef_st/2
  VCU1_TorqueRef_st/1 -> VCU1_TorqueRef_D/1
  VCU1_TorqueRef_F/1 -> VCU1_TorqueRef_D/2
  VCU1_TorqueRef_D/1 -> VCU1_TorqueRefRon/1
  VCU1_TorqueRefRon/1 -> VCU1_TorqueRef_S/1
  VCU1_TorqueRef_S/1 -> VCU1_TorqueRef_1sat/1
  VCU1_TorqueRef_1sat/1 -> VCU1_TorqueRef_Convert/1
  VCU1_TorqueRef_Convert/1 -> VCU1_TorqueRef_L/1
  VCU1_TorqueRef_L/1 -> VCU1_TorqueRef_D1/1, VCU1_TorqueRef_And/1
  VCU1_TorqueRefoutput4_C/1 -> VCU1_TorqueRef_D1/2
  VCU1_TorqueRef_D1/1 -> VCU1_TorqueRefCOV/1
  VCU1_TorqueRefCOV/1 -> output4/1
  VCU1_TorqueRef_And_C/1 -> VCU1_TorqueRef_And/2
  VCU1_TorqueRef_And/1 -> VCU1_TorqueRefBitCov/1
  VCU1_TorqueRefBitCov/1 -> output5/1
  Constant1/1 -> output1/1
  Constant2/1 -> output2/1
  Constant3/1 -> output3/1
  Constant6/1 -> output6/1
  Constant7/1 -> output7/1
  Constant8/1 -> output8/1

== system six_plus_six_AcmsteeringV09_main/Subsystem/VCU3/VCU1_CtrlModel ==
  VCU1_CtrlModel : Inport
  Constant{2..8} (7 alike) : Constant  Value=0  OutDataTypeStr=uint8
  VCU1_CtrlModelRon : Rounding  Operator=round
  VCU1_CtrlModel_1sat : Saturate  UpperLimit=4  LowerLimit=0
  VCU1_CtrlModel_Convert : DataTypeConversion  OutDataTypeStr=uint8
  VCU1_CtrlModel_Convert1 : DataTypeConversion  OutDataTypeStr=uint32
  VCU1_CtrlModel_D : Product  Inputs=*/
  VCU1_CtrlModel_F : Constant  OutDataTypeStr=single
  VCU1_CtrlModel_L : simulink/Logic and Bit Operations/Bitwise Operator  logicop=AND  UseBitMask=on  BitMask=4  BitMaskRealWorld=Stored Integer
  VCU1_CtrlModel_O : Constant  Value=0  OutDataTypeStr=single
  VCU1_CtrlModel_S : ArithShift  BitShiftNumber=-2
  VCU1_CtrlModel_sat : Saturate  UpperLimit=1  LowerLimit=0
  VCU1_CtrlModel_st : Sum  Inputs=+-
  output1 : Outport
  output2 : Outport  Port=2
  output3 : Outport  Port=3
  output4 : Outport  Port=4
  output5 : Outport  Port=5
  output6 : Outport  Port=6
  output7 : Outport  Port=7
  output8 : Outport  Port=8
  wires:
  VCU1_CtrlModel/1 -> VCU1_CtrlModel_sat/1
  VCU1_CtrlModel_sat/1 -> VCU1_CtrlModel_st/1
  VCU1_CtrlModel_O/1 -> VCU1_CtrlModel_st/2
  VCU1_CtrlModel_st/1 -> VCU1_CtrlModel_D/1
  VCU1_CtrlModel_F/1 -> VCU1_CtrlModel_D/2
  VCU1_CtrlModel_D/1 -> VCU1_CtrlModelRon/1
  VCU1_CtrlModelRon/1 -> VCU1_CtrlModel_S/1
  VCU1_CtrlModel_S/1 -> VCU1_CtrlModel_1sat/1
  VCU1_CtrlModel_1sat/1 -> VCU1_CtrlModel_Convert1/1
  VCU1_CtrlModel_Convert1/1 -> VCU1_CtrlModel_L/1
  VCU1_CtrlModel_L/1 -> VCU1_CtrlModel_Convert/1
  VCU1_CtrlModel_Convert/1 -> output1/1
  Constant2/1 -> output2/1
  Constant3/1 -> output3/1
  Constant4/1 -> output4/1
  Constant5/1 -> output5/1
  Constant6/1 -> output6/1
  Constant7/1 -> output7/1
  Constant8/1 -> output8/1

== system six_plus_six_AcmsteeringV09_main/Subsystem/VCU3/VCU1_EnableReq ==
  VCU1_EnableReq : Inport
  Constant{2..8} (7 alike) : Constant  Value=0  OutDataTypeStr=uint8
  VCU1_EnableReqRon : Rounding  Operator=round
  VCU1_EnableReq_1sat : Saturate  UpperLimit=3  LowerLimit=0
  VCU1_EnableReq_Convert : DataTypeConversion  OutDataTypeStr=uint8
  VCU1_EnableReq_Convert1 : DataTypeConversion  OutDataTypeStr=uint32
  VCU1_EnableReq_D : Product  Inputs=*/
  VCU1_EnableReq_F : Constant  OutDataTypeStr=single
  VCU1_EnableReq_L : simulink/Logic and Bit Operations/Bitwise Operator  logicop=AND  UseBitMask=on  BitMask=3  BitMaskRealWorld=Stored Integer
  VCU1_EnableReq_O : Constant  Value=0  OutDataTypeStr=single
  VCU1_EnableReq_S : ArithShift
  VCU1_EnableReq_sat : Saturate  UpperLimit=3  LowerLimit=0
  VCU1_EnableReq_st : Sum  Inputs=+-
  output1 : Outport
  output2 : Outport  Port=2
  output3 : Outport  Port=3
  output4 : Outport  Port=4
  output5 : Outport  Port=5
  output6 : Outport  Port=6
  output7 : Outport  Port=7
  output8 : Outport  Port=8
  wires:
  VCU1_EnableReq/1 -> VCU1_EnableReq_sat/1
  VCU1_EnableReq_sat/1 -> VCU1_EnableReq_st/1
  VCU1_EnableReq_O/1 -> VCU1_EnableReq_st/2
  VCU1_EnableReq_st/1 -> VCU1_EnableReq_D/1
  VCU1_EnableReq_F/1 -> VCU1_EnableReq_D/2
  VCU1_EnableReq_D/1 -> VCU1_EnableReqRon/1
  VCU1_EnableReqRon/1 -> VCU1_EnableReq_S/1
  VCU1_EnableReq_S/1 -> VCU1_EnableReq_1sat/1
  VCU1_EnableReq_1sat/1 -> VCU1_EnableReq_Convert1/1
  VCU1_EnableReq_Convert1/1 -> VCU1_EnableReq_L/1
  VCU1_EnableReq_L/1 -> VCU1_EnableReq_Convert/1
  VCU1_EnableReq_Convert/1 -> output1/1
  Constant2/1 -> output2/1
  Constant3/1 -> output3/1
  Constant4/1 -> output4/1
  Constant5/1 -> output5/1
  Constant6/1 -> output6/1
  Constant7/1 -> output7/1
  Constant8/1 -> output8/1

== system six_plus_six_AcmsteeringV09_main/Subsystem/VCU3/VCU1_GearCmd ==
  VCU1_GearCmd : Inport
  Constant{2..8} (7 alike) : Constant  Value=0  OutDataTypeStr=uint8
  VCU1_GearCmdRon : Rounding  Operator=round
  VCU1_GearCmd_1sat : Saturate  UpperLimit=24  LowerLimit=0
  VCU1_GearCmd_Convert : DataTypeConversion  OutDataTypeStr=uint8
  VCU1_GearCmd_Convert1 : DataTypeConversion  OutDataTypeStr=uint32
  VCU1_GearCmd_D : Product  Inputs=*/
  VCU1_GearCmd_F : Constant  OutDataTypeStr=single
  VCU1_GearCmd_L : simulink/Logic and Bit Operations/Bitwise Operator  logicop=AND  UseBitMask=on  BitMask=24  BitMaskRealWorld=Stored Integer
  VCU1_GearCmd_O : Constant  Value=0  OutDataTypeStr=single
  VCU1_GearCmd_S : ArithShift  BitShiftNumber=-3
  VCU1_GearCmd_sat : Saturate  UpperLimit=3  LowerLimit=0
  VCU1_GearCmd_st : Sum  Inputs=+-
  output1 : Outport
  output2 : Outport  Port=2
  output3 : Outport  Port=3
  output4 : Outport  Port=4
  output5 : Outport  Port=5
  output6 : Outport  Port=6
  output7 : Outport  Port=7
  output8 : Outport  Port=8
  wires:
  VCU1_GearCmd/1 -> VCU1_GearCmd_sat/1
  VCU1_GearCmd_sat/1 -> VCU1_GearCmd_st/1
  VCU1_GearCmd_O/1 -> VCU1_GearCmd_st/2
  VCU1_GearCmd_st/1 -> VCU1_GearCmd_D/1
  VCU1_GearCmd_F/1 -> VCU1_GearCmd_D/2
  VCU1_GearCmd_D/1 -> VCU1_GearCmdRon/1
  VCU1_GearCmdRon/1 -> VCU1_GearCmd_S/1
  VCU1_GearCmd_S/1 -> VCU1_GearCmd_1sat/1
  VCU1_GearCmd_1sat/1 -> VCU1_GearCmd_Convert1/1
  VCU1_GearCmd_Convert1/1 -> VCU1_GearCmd_L/1
  VCU1_GearCmd_L/1 -> VCU1_GearCmd_Convert/1
  VCU1_GearCmd_Convert/1 -> output1/1
  Constant2/1 -> output2/1
  Constant3/1 -> output3/1
  Constant4/1 -> output4/1
  Constant5/1 -> output5/1
  Constant6/1 -> output6/1
  Constant7/1 -> output7/1
  Constant8/1 -> output8/1

== system six_plus_six_AcmsteeringV09_main/Subsystem/VCU3/VCU1_LifeCnt ==
  VCU1_LifeCnt : Inport
  Constant{1..7} (7 alike) : Constant  Value=0  OutDataTypeStr=uint8
  VCU1_LifeCntRon : Rounding  Operator=round
  VCU1_LifeCnt_1sat : Saturate  UpperLimit=255  LowerLimit=0
  VCU1_LifeCnt_Convert : DataTypeConversion  OutDataTypeStr=uint8
  VCU1_LifeCnt_Convert1 : DataTypeConversion  OutDataTypeStr=uint32
  VCU1_LifeCnt_D : Product  Inputs=*/
  VCU1_LifeCnt_F : Constant  OutDataTypeStr=single
  VCU1_LifeCnt_L : simulink/Logic and Bit Operations/Bitwise Operator  logicop=AND  UseBitMask=on  BitMask=255  BitMaskRealWorld=Stored Integer
  VCU1_LifeCnt_O : Constant  Value=0  OutDataTypeStr=single
  VCU1_LifeCnt_S : ArithShift
  VCU1_LifeCnt_sat : Saturate  UpperLimit=255  LowerLimit=0
  VCU1_LifeCnt_st : Sum  Inputs=+-
  output1 : Outport
  output2 : Outport  Port=2
  output3 : Outport  Port=3
  output4 : Outport  Port=4
  output5 : Outport  Port=5
  output6 : Outport  Port=6
  output7 : Outport  Port=7
  output8 : Outport  Port=8
  wires:
  VCU1_LifeCnt/1 -> VCU1_LifeCnt_sat/1
  VCU1_LifeCnt_sat/1 -> VCU1_LifeCnt_st/1
  VCU1_LifeCnt_O/1 -> VCU1_LifeCnt_st/2
  VCU1_LifeCnt_st/1 -> VCU1_LifeCnt_D/1
  VCU1_LifeCnt_F/1 -> VCU1_LifeCnt_D/2
  VCU1_LifeCnt_D/1 -> VCU1_LifeCntRon/1
  VCU1_LifeCntRon/1 -> VCU1_LifeCnt_S/1
  VCU1_LifeCnt_S/1 -> VCU1_LifeCnt_1sat/1
  VCU1_LifeCnt_1sat/1 -> VCU1_LifeCnt_Convert1/1
  VCU1_LifeCnt_Convert1/1 -> VCU1_LifeCnt_L/1
  VCU1_LifeCnt_L/1 -> VCU1_LifeCnt_Convert/1
  VCU1_LifeCnt_Convert/1 -> output8/1
  Constant1/1 -> output1/1
  Constant2/1 -> output2/1
  Constant3/1 -> output3/1
  Constant4/1 -> output4/1
  Constant5/1 -> output5/1
  Constant6/1 -> output6/1
  Constant7/1 -> output7/1

== system six_plus_six_AcmsteeringV09_main/Subsystem/VCU3/VCU1_SpeedMax ==
  VCU1_SpeedMax : Inport
  Constant{1,4..8} (6 alike) : Constant  Value=0  OutDataTypeStr=uint8
  VCU1_SpeedMaxBitCov : DataTypeConversion  OutDataTypeStr=uint8
  VCU1_SpeedMaxCOV : DataTypeConversion  OutDataTypeStr=uint8
  VCU1_SpeedMaxRon : Rounding  Operator=round
  VCU1_SpeedMax_1sat : Saturate  UpperLimit=65535  LowerLimit=0
  VCU1_SpeedMax_And : simulink/Logic and Bit Operations/Bitwise Operator  logicop=AND  UseBitMask=off  NumInputPorts=2  BitMask=bin2dec('11011001')  BitMaskRealWorld=Stored Integer
  VCU1_SpeedMax_And_C : Constant  Value=255  OutDataTypeStr=uint32
  VCU1_SpeedMax_Convert : DataTypeConversion  OutDataTypeStr=uint32
  VCU1_SpeedMax_D : Product  Inputs=*/
  VCU1_SpeedMax_D1 : Product  Inputs=*/
  VCU1_SpeedMax_F : Constant  OutDataTypeStr=single
  VCU1_SpeedMax_L : simulink/Logic and Bit Operations/Bitwise Operator  logicop=AND  UseBitMask=on  BitMask=65535  BitMaskRealWorld=Stored Integer
  VCU1_SpeedMax_O : Constant  Value=0  OutDataTypeStr=single
  VCU1_SpeedMax_S : ArithShift
  VCU1_SpeedMax_sat : Saturate  UpperLimit=10000  LowerLimit=0
  VCU1_SpeedMax_st : Sum  Inputs=+-
  VCU1_SpeedMaxoutput2_C : Constant  Value=256
  output1 : Outport
  output2 : Outport  Port=2
  output3 : Outport  Port=3
  output4 : Outport  Port=4
  output5 : Outport  Port=5
  output6 : Outport  Port=6
  output7 : Outport  Port=7
  output8 : Outport  Port=8
  wires:
  VCU1_SpeedMax/1 -> VCU1_SpeedMax_sat/1
  VCU1_SpeedMax_sat/1 -> VCU1_SpeedMax_st/1
  VCU1_SpeedMax_O/1 -> VCU1_SpeedMax_st/2
  VCU1_SpeedMax_st/1 -> VCU1_SpeedMax_D/1
  VCU1_SpeedMax_F/1 -> VCU1_SpeedMax_D/2
  VCU1_SpeedMax_D/1 -> VCU1_SpeedMaxRon/1
  VCU1_SpeedMaxRon/1 -> VCU1_SpeedMax_S/1
  VCU1_SpeedMax_S/1 -> VCU1_SpeedMax_1sat/1
  VCU1_SpeedMax_1sat/1 -> VCU1_SpeedMax_Convert/1
  VCU1_SpeedMax_Convert/1 -> VCU1_SpeedMax_L/1
  VCU1_SpeedMax_L/1 -> VCU1_SpeedMax_D1/1, VCU1_SpeedMax_And/1
  VCU1_SpeedMaxoutput2_C/1 -> VCU1_SpeedMax_D1/2
  VCU1_SpeedMax_D1/1 -> VCU1_SpeedMaxCOV/1
  VCU1_SpeedMaxCOV/1 -> output2/1
  VCU1_SpeedMax_And_C/1 -> VCU1_SpeedMax_And/2
  VCU1_SpeedMax_And/1 -> VCU1_SpeedMaxBitCov/1
  VCU1_SpeedMaxBitCov/1 -> output3/1
  Constant1/1 -> output1/1
  Constant4/1 -> output4/1
  Constant5/1 -> output5/1
  Constant6/1 -> output6/1
  Constant7/1 -> output7/1
  Constant8/1 -> output8/1

== matlab function six_plus_six_AcmsteeringV09_main/MainControl/mode_control/forward/forward/Brake/Switch Case Action Subsystem/MATLAB Function5 ==
  data: bratrq_dem_lf input; bratrq_dem_lm input; bratrq_dem_lr input; bratrq_dem_rf input; bratrq_dem_rm input; bratrq_dem_rr input; pwr_chg_bat input; bratrq_mot_lf output; bratrq_mot_lm output; pwr_chg_bat1 input; pwr_chg_bat2 input; trqlimL_dig_lf input; bratrq_mot_lr output; bratrq_mot_rf output; bratrq_mot_rm output; bratrq_mot_rr output; trqlimL_dig_lm input; trqlimL_dig_lr input; trqlimL_dig_rf input; trqlimL_dig_rm input; trqlimL_dig_rr input; speed_act_lf input; speed_act_lm input; speed_act_lr input; speed_act_rf input; speed_act_rm input; speed_act_rr input; trqlim_map_lf input; brapre_out_l output; brapre_out_r output; trqlim_map_lm input; trqlim_map_lr input; trqlim_map_rf input; trqlim_map_rm input; trqlim_map_rr input; tras_ratio input; guzhang_lf input; guzhang_lm input; guzhang_lr input; guzhang_rf input; guzhang_rm input; guzhang_rr input
function [bratrq_mot_lf,bratrq_mot_lm,bratrq_mot_lr,bratrq_mot_rf,bratrq_mot_rm,bratrq_mot_rr,brapre_out_l,brapre_out_r] = fcn(bratrq_dem_lf,bratrq_dem_lm,bratrq_dem_lr,bratrq_dem_rf,bratrq_dem_rm,bratrq_dem_rr,pwr_chg_bat,pwr_chg_bat1,pwr_chg_bat2,trqlimL_dig_lf,trqlimL_dig_lm,trqlimL_dig_lr,trqlimL_dig_rf,trqlimL_dig_rm,trqlimL_dig_rr,speed_act_lf,speed_act_lm,speed_act_lr,speed_act_rf,speed_act_rm,speed_act_rr,trqlim_map_lf,trqlim_map_lm,trqlim_map_lr,trqlim_map_rf,trqlim_map_rm,trqlim_map_rr,tras_ratio,guzhang_lf,guzhang_lm,guzhang_lr,guzhang_rf,guzhang_rm,guzhang_rr)
%#codegen pid模块在外面做，里面进行十六种情况的判断，先看一下效果，不能再修改。前轴单独控制，后轴低选控制

bratrq_mot_lf1=single(bratrq_dem_lf/tras_ratio);
bratrq_mot_lf2=single(9549*(pwr_chg_bat/2)/speed_act_lf);
bratrq_mot_lf=single(min(trqlimL_dig_lf,min(bratrq_mot_lf1,bratrq_mot_lf2)));

bratrq_mot_lm1=single(bratrq_dem_lm/tras_ratio);
bratrq_mot_lm2=single(9549*(pwr_chg_bat1/2)/speed_act_lm);
bratrq_mot_lm=single(min(trqlimL_dig_lm,min(bratrq_mot_lm1,bratrq_mot_lm2)));

bratrq_mot_lr1=single(bratrq_dem_lr/tras_ratio);
bratrq_mot_lr2=single(9549*(pwr_chg_bat2/2)/speed_act_lr);
bratrq_mot_lr=single(min(trqlimL_dig_lr,min(bratrq_mot_lr1,bratrq_mot_lr2)));
 
bratrq_mot_rf1=single(bratrq_dem_rf/tras_ratio);
bratrq_mot_rf2=single(9549*(pwr_chg_bat/2)/speed_act_rf);
bratrq_mot_rf=single(min(trqlimL_dig_rf,min(bratrq_mot_rf1,bratrq_mot_rf2)));

bratrq_mot_rm1=single(bratrq_dem_rm/tras_ratio);
bratrq_mot_rm2=single(9549*(pwr_chg_bat1/2)/speed_act_rm);
bratrq_mot_rm=single(min(trqlimL_dig_rm,min(bratrq_mot_rm1,bratrq_mot_rm2)));

bratrq_mot_rr1=single(bratrq_dem_rr/tras_ratio);
bratrq_mot_rr2=single(9549*(pwr_chg_bat2/2)/speed_act_rr);
bratrq_mot_rr=single(min(trqlimL_dig_rr,min(bratrq_mot_rr1,bratrq_mot_rr2)));

brapre_out_l=single(((bratrq_dem_lf+bratrq_dem_lm+bratrq_dem_lr)-(bratrq_mot_lf+bratrq_mot_lm+bratrq_mot_lr)*tras_ratio)/3/150);
brapre_out_r=single(((bratrq_dem_rf+bratrq_dem_rm+bratrq_dem_rr)-(bratrq_mot_rf+bratrq_mot_rm+bratrq_mot_rr)*tras_ratio)/3/150);







bratrq_mot_lf=single(min(bratrq_mot_lf,trqlim_map_lf));%限一下最大值在外特性内，最小值大于0
bratrq_mot_lf=single(max(bratrq_mot_lf,0));
bratrq_mot_lr=single(min(bratrq_mot_lr,trqlim_map_lr));
bratrq_mot_lr=single(max(bratrq_mot_lr,0));
bratrq_mot_rf=single(min(bratrq_mot_rf,trqlim_map_rf));
bratrq_mot_rf=single(max(bratrq_mot_rf,0));
bratrq_mot_rr=single(min(bratrq_mot_rr,trqlim_map_rr));
bratrq_mot_rr=single(max(bratrq_mot_rr,0));

% brapre_out_l=brapre_out_l;
% brapre_out_r=brapre_out_r;
brapre_out_l=single(brapre_out_l*150/125);%第二辆车的制动压力与制动力的关系调整一下。
brapre_out_r=single(brapre_out_r*150/125);

if guzhang_lf==1
    bratrq_mot_lf=single(0);
end
if guzhang_lm==1
    bratrq_mot_lm=single(0);
end
if guzhang_lr==1
    bratrq_mot_lr=single(0);
end
if guzhang_rf==1
    bratrq_mot_rf=single(0);
end
if guzhang_rm==1
    bratrq_mot_rm=single(0);
end
if guzhang_rr==1
    bratrq_mot_rr=single(0);
end

end

== system six_plus_six_AcmsteeringV09_main/Subsystem/VCU3/VCU1_TorqueRef ==
  VCU1_TorqueRef : Inport
  Constant{1..3,6..8} (6 alike) : Constant  Value=0  OutDataTypeStr=uint8
  VCU1_TorqueRefBitCov : DataTypeConversion  OutDataTypeStr=uint8
  VCU1_TorqueRefCOV : DataTypeConversion  OutDataTypeStr=uint8
  VCU1_TorqueRefRon : Rounding  Operator=round
  VCU1_TorqueRef_1sat : Saturate  UpperLimit=65535  LowerLimit=0
  VCU1_TorqueRef_And : simulink/Logic and Bit Operations/Bitwise Operator  logicop=AND  UseBitMask=off  NumInputPorts=2  BitMask=bin2dec('11011001')  BitMaskRealWorld=Stored Integer
  VCU1_TorqueRef_And_C : Constant  Value=255  OutDataTypeStr=uint32
  VCU1_TorqueRef_Convert : DataTypeConversion  OutDataTypeStr=uint32
  VCU1_TorqueRef_D : Product  Inputs=*/
  VCU1_TorqueRef_D1 : Product  Inputs=*/
  VCU1_TorqueRef_F : Constant  Value=0.1  OutDataTypeStr=single
  VCU1_TorqueRef_L : simulink/Logic and Bit Operations/Bitwise Operator  logicop=AND  UseBitMask=on  BitMask=65535  BitMaskRealWorld=Stored Integer
  VCU1_TorqueRef_O : Constant  Value=-1000  OutDataTypeStr=single
  VCU1_TorqueRef_S : ArithShift
  VCU1_TorqueRef_sat : Saturate  UpperLimit=1000  LowerLimit=-1000
  VCU1_TorqueRef_st : Sum  Inputs=+-
  VCU1_TorqueRefoutput4_C : Constant  Value=256
  output1 : Outport
  output2 : Outport  Port=2
  output3 : Outport  Port=3
  output4 : Outport  Port=4
  output5 : Outport  Port=5
  output6 : Outport  Port=6
  output7 : Outport  Port=7
  output8 : Outport  Port=8
  wires:
  VCU1_TorqueRef/1 -> VCU1_TorqueRef_sat/1
  VCU1_TorqueRef_sat/1 -> VCU1_TorqueRef_st/1
  VCU1_TorqueRef_O/1 -> VCU1_TorqueRef_st/2
  VCU1_TorqueRef_st/1 -> VCU1_TorqueRef_D/1
  VCU1_TorqueRef_F/1 -> VCU1_TorqueRef_D/2
  VCU1_TorqueRef_D/1 -> VCU1_TorqueRefRon/1
  VCU1_TorqueRefRon/1 -> VCU1_TorqueRef_S/1
  VCU1_TorqueRef_S/1 -> VCU1_TorqueRef_1sat/1
  VCU1_TorqueRef_1sat/1 -> VCU1_TorqueRef_Convert/1
  VCU1_TorqueRef_Convert/1 -> VCU1_TorqueRef_L/1
  VCU1_TorqueRef_L/1 -> VCU1_TorqueRef_D1/1, VCU1_TorqueRef_And/1
  VCU1_TorqueRefoutput4_C/1 -> VCU1_TorqueRef_D1/2
  VCU1_TorqueRef_D1/1 -> VCU1_TorqueRefCOV/1
  VCU1_TorqueRefCOV/1 -> output4/1
  VCU1_TorqueRef_And_C/1 -> VCU1_TorqueRef_And/2
  VCU1_TorqueRef_And/1 -> VCU1_TorqueRefBitCov/1
  VCU1_TorqueRefBitCov/1 -> output5/1
  Constant1/1 -> output1/1
  Constant2/1 -> output2/1
  Constant3/1 -> output3/1
  Constant6/1 -> output6/1
  Constant7/1 -> output7/1
  Constant8/1 -> output8/1

== system six_plus_six_AcmsteeringV09_main/Subsystem/VCU4/VCU1_CtrlModel ==
  VCU1_CtrlModel : Inport
  Constant{2..8} (7 alike) : Constant  Value=0  OutDataTypeStr=uint8
  VCU1_CtrlModelRon : Rounding  Operator=round
  VCU1_CtrlModel_1sat : Saturate  UpperLimit=4  LowerLimit=0
  VCU1_CtrlModel_Convert : DataTypeConversion  OutDataTypeStr=uint8
  VCU1_CtrlModel_Convert1 : DataTypeConversion  OutDataTypeStr=uint32
  VCU1_CtrlModel_D : Product  Inputs=*/
  VCU1_CtrlModel_F : Constant  OutDataTypeStr=single
  VCU1_CtrlModel_L : simulink/Logic and Bit Operations/Bitwise Operator  logicop=AND  UseBitMask=on  BitMask=4  BitMaskRealWorld=Stored Integer
  VCU1_CtrlModel_O : Constant  Value=0  OutDataTypeStr=single
  VCU1_CtrlModel_S : ArithShift  BitShiftNumber=-2
  VCU1_CtrlModel_sat : Saturate  UpperLimit=1  LowerLimit=0
  VCU1_CtrlModel_st : Sum  Inputs=+-
  output1 : Outport
  output2 : Outport  Port=2
  output3 : Outport  Port=3
  output4 : Outport  Port=4
  output5 : Outport  Port=5
  output6 : Outport  Port=6
  output7 : Outport  Port=7
  output8 : Outport  Port=8
  wires:
  VCU1_CtrlModel/1 -> VCU1_CtrlModel_sat/1
  VCU1_CtrlModel_sat/1 -> VCU1_CtrlModel_st/1
  VCU1_CtrlModel_O/1 -> VCU1_CtrlModel_st/2
  VCU1_CtrlModel_st/1 -> VCU1_CtrlModel_D/1
  VCU1_CtrlModel_F/1 -> VCU1_CtrlModel_D/2
  VCU1_CtrlModel_D/1 -> VCU1_CtrlModelRon/1
  VCU1_CtrlModelRon/1 -> VCU1_CtrlModel_S/1
  VCU1_CtrlModel_S/1 -> VCU1_CtrlModel_1sat/1
  VCU1_CtrlModel_1sat/1 -> VCU1_CtrlModel_Convert1/1
  VCU1_CtrlModel_Convert1/1 -> VCU1_CtrlModel_L/1
  VCU1_CtrlModel_L/1 -> VCU1_CtrlModel_Convert/1
  VCU1_CtrlModel_Convert/1 -> output1/1
  Constant2/1 -> output2/1
  Constant3/1 -> output3/1
  Constant4/1 -> output4/1
  Constant5/1 -> output5/1
  Constant6/1 -> output6/1
  Constant7/1 -> output7/1
  Constant8/1 -> output8/1

== system six_plus_six_AcmsteeringV09_main/Subsystem/VCU4/VCU1_EnableReq ==
  VCU1_EnableReq : Inport
  Constant{2..8} (7 alike) : Constant  Value=0  OutDataTypeStr=uint8
  VCU1_EnableReqRon : Rounding  Operator=round
  VCU1_EnableReq_1sat : Saturate  UpperLimit=3  LowerLimit=0
  VCU1_EnableReq_Convert : DataTypeConversion  OutDataTypeStr=uint8
  VCU1_EnableReq_Convert1 : DataTypeConversion  OutDataTypeStr=uint32
  VCU1_EnableReq_D : Product  Inputs=*/
  VCU1_EnableReq_F : Constant  OutDataTypeStr=single
  VCU1_EnableReq_L : simulink/Logic and Bit Operations/Bitwise Operator  logicop=AND  UseBitMask=on  BitMask=3  BitMaskRealWorld=Stored Integer
  VCU1_EnableReq_O : Constant  Value=0  OutDataTypeStr=single
  VCU1_EnableReq_S : ArithShift
  VCU1_EnableReq_sat : Saturate  UpperLimit=3  LowerLimit=0
  VCU1_EnableReq_st : Sum  Inputs=+-
  output1 : Outport
  output2 : Outport  Port=2
  output3 : Outport  Port=3
  output4 : Outport  Port=4
  output5 : Outport  Port=5
  output6 : Outport  Port=6
  output7 : Outport  Port=7
  output8 : Outport  Port=8
  wires:
  VCU1_EnableReq/1 -> VCU1_EnableReq_sat/1
  VCU1_EnableReq_sat/1 -> VCU1_EnableReq_st/1
  VCU1_EnableReq_O/1 -> VCU1_EnableReq_st/2
  VCU1_EnableReq_st/1 -> VCU1_EnableReq_D/1
  VCU1_EnableReq_F/1 -> VCU1_EnableReq_D/2
  VCU1_EnableReq_D/1 -> VCU1_EnableReqRon/1
  VCU1_EnableReqRon/1 -> VCU1_EnableReq_S/1
  VCU1_EnableReq_S/1 -> VCU1_EnableReq_1sat/1
  VCU1_EnableReq_1sat/1 -> VCU1_EnableReq_Convert1/1
  VCU1_EnableReq_Convert1/1 -> VCU1_EnableReq_L/1
  VCU1_EnableReq_L/1 -> VCU1_EnableReq_Convert/1
  VCU1_EnableReq_Convert/1 -> output1/1
  Constant2/1 -> output2/1
  Constant3/1 -> output3/1
  Constant4/1 -> output4/1
  Constant5/1 -> output5/1
  Constant6/1 -> output6/1
  Constant7/1 -> output7/1
  Constant8/1 -> output8/1
